simulink model "part1_2024a_Audun"  (R2024a)
settings: Solver=VariableStepAuto  StartTime=0.0  StopTime=50  RelTol=1e-3
undefined symbols (not defined in the file or in its folder): alpha, C_pitch, C_roll, C_yaw, Cx, Cy, Cz, Hoerner, magnitude, thrusters, vessel
libraries: marine_gnc x3, marine_hydro x1, simulink x1
settings Model: Creator=jonbjor  LastModifiedBy=audun
settings SolverCC: AlgebraicLoopSolver=TrustRegion
settings DataIOCC: ReturnWorkspaceOutputs=off
settings DebuggingCC: UnconnectedInputMsg=warning  UnconnectedOutputMsg=warning  UnconnectedLineMsg=warning  ArithmeticOperatorsInVariantConditions=warning
settings ModelReferenceCC: EnableRefExpFcnMdlSchedulingChecks=on
settings SFSimCC: SimUseLocalCustomCode=off  CustomCodeUndefinedFunction=UseInterfaceOnly
settings RTWCC: RTWUseLocalCustomCode=off  GPUComputeCapability=3.5  DLArmComputeVersion=19.05

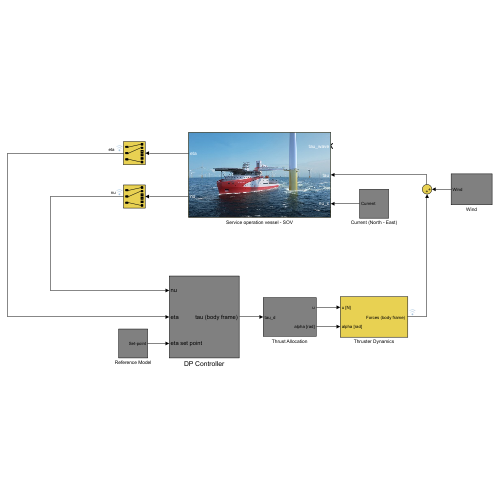
[thumbnail: Simulink's stored preview of the top-level diagram]
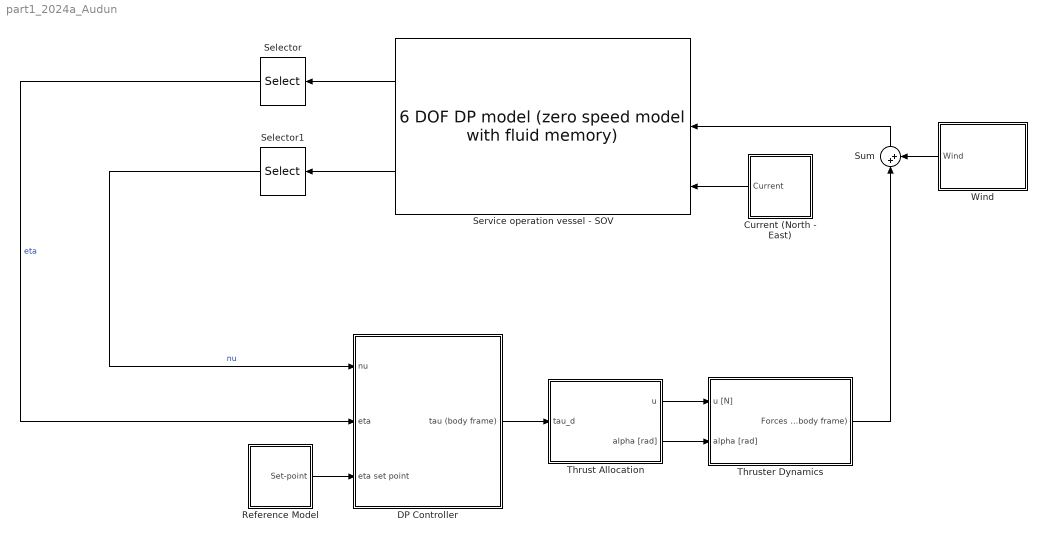
== system part1_2024a_Audun ==
  Current (North - East) : Subsystem
  DP Controller : Subsystem
  Reference Model : Subsystem
  Selector : Selector  InputPortWidth=6  IndexOptions=Index vector (dialog)  Indices=[1 2 6]  OutputSizes=1
  Selector1 : Selector  InputPortWidth=6  IndexOptions=Index vector (dialog)  Indices=[1 2 6]  OutputSizes=1
  Service operation vessel - SOV : marine_hydro/Hydro Library/6 DOF DP model  (zero speed model with fluid memory)  ABC=vesselABC  rho=1025  Axc=0.9*vessel.main.T*vessel.main.B  Ayc=0.9*vessel.main.T*vessel.main.Lpp  CX=1  CY_2D=Hoerner(vessel.main.B,vessel.main.T)  Bv=vessel.Bv  mask(6 DOF zero speed model){}
      link override "Integrator1 ": InitialCondition=nu0
      link override Integrator2: InitialCondition=eta0
      settings: SourceProductName=MSS Hydro
      mask Display:
      | image('SOV.jpg');
      | color('white'); port_label('output', 1, 'eta')
      | color('white'); port_label('output', 2, 'nu')
      | color('white'); port_label('input', 1, 'tau_wave')
      | color('white'); port_label('input', 2, 'tau')
      | color('white'); port_label('input', 3, 'nu_c')
  Sum : Sum  Inputs=|++
  Thrust Allocation : Subsystem
  Thruster Dynamics : Subsystem  mask{thrusterfault=off}
      mask prompts: thrusterfault "Fault on thruster #2 and #4?"
  Wind : Subsystem
  wires:
  Current (North - East)/1(Current) -> Service operation vessel - SOV/3
  Thruster Dynamics/1("Forces (body frame) ") -> Sum/1
  Service operation vessel - SOV/1 -> Selector/1
  Service operation vessel - SOV/2 -> Selector1/1
  Reference Model/1(Set-point) -> DP Controller/3(eta set point)
  Selector/1 -> DP Controller/2(eta)  "eta"
  Selector1/1 -> DP Controller/1(nu)  "nu"
  Thrust Allocation/1(u) -> Thruster Dynamics/1(u [N])
  Thrust Allocation/2(alpha [rad]) -> Thruster Dynamics/2(alpha [rad])
  DP Controller/1(tau (body frame)) -> Thrust Allocation/1(tau_d)
  Wind/1(Wind) -> Sum/2
  Sum/1 -> Service operation vessel - SOV/2

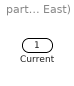
== system part1_2024a_Audun/Current (North - East) ==
  Current : Outport  VectorParamsAs1DForOutWhenUnconnected=off

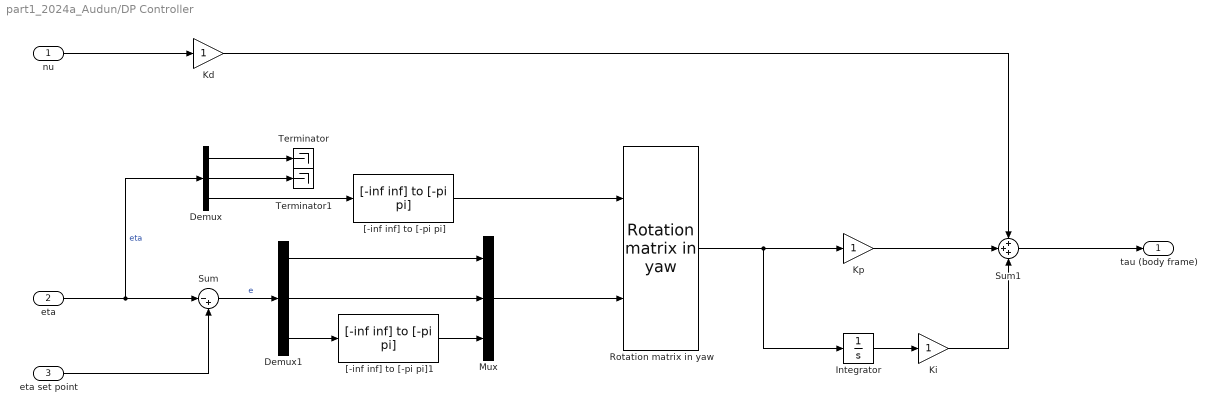
== system part1_2024a_Audun/DP Controller ==
  nu : Inport
  eta : Inport  Port=2
  eta set point : Inport  Port=3
  Demux : Demux  Outputs=3
  Demux1 : Demux  Outputs=3
  Integrator : Integrator
  Kd : Gain
  Ki : Gain
  Kp : Gain
  Mux : Mux  Inputs=3
  "Rotation matrix in yaw " : marine_gnc/Models/ Kinematics/Rotation matrix in yaw 
      settings: SourceProductName=MSS GNC
  Sum : Sum  Inputs=|-+
  Sum1 : Sum  Inputs=+++
  Terminator : Terminator
  Terminator1 : Terminator
  "[-inf inf] to [-pi pi]" : marine_gnc/Utilities/Math Operations/[-inf inf] to [-pi pi]
      settings: SourceProductName=MSS GNC
  "[-inf inf] to [-pi pi]1" : marine_gnc/Utilities/Math Operations/[-inf inf] to [-pi pi]
      settings: SourceProductName=MSS GNC
  tau (body frame) : Outport  VectorParamsAs1DForOutWhenUnconnected=off
  wires:
  eta set point/1 -> Sum/2
  eta/1 -> Demux/1, Sum/1  "eta"
  Sum/1 -> Demux1/1  "e"
  nu/1 -> Kd/1
  Demux/1 -> Terminator/1
  Demux/2 -> Terminator1/1
  Demux/3 -> "[-inf inf] to [-pi pi]"/1
  "[-inf inf] to [-pi pi]"/1 -> "Rotation matrix in yaw "/1
  Demux1/2 -> Mux/2
  Demux1/3 -> "[-inf inf] to [-pi pi]1"/1
  Demux1/1 -> Mux/1
  Mux/1 -> "Rotation matrix in yaw "/2
  "[-inf inf] to [-pi pi]1"/1 -> Mux/3
  "Rotation matrix in yaw "/1 -> Integrator/1, Kp/1
  Integrator/1 -> Ki/1
  Ki/1 -> Sum1/3
  Kp/1 -> Sum1/2
  Kd/1 -> Sum1/1
  Sum1/1 -> tau (body frame)/1

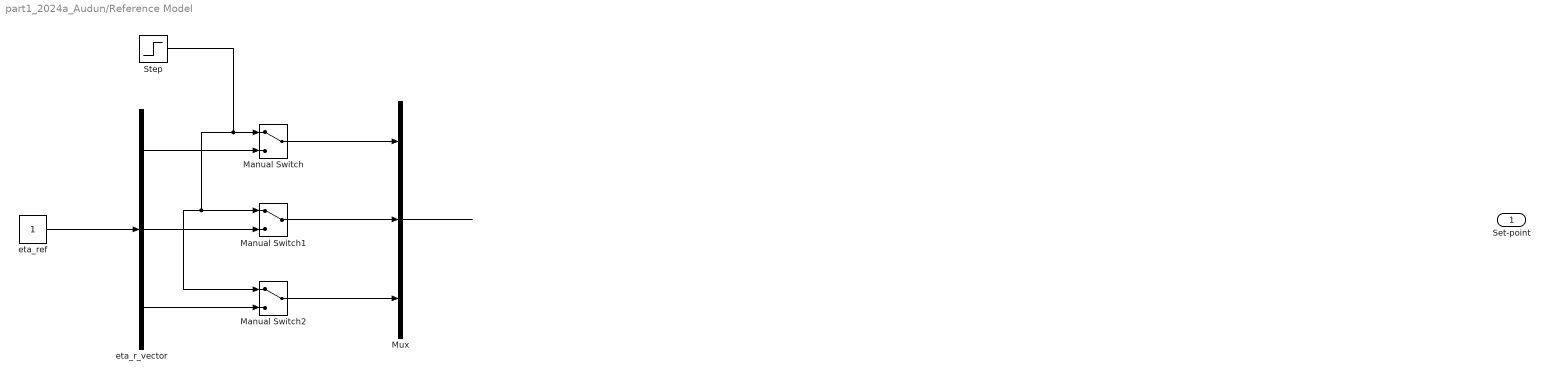
== system part1_2024a_Audun/Reference Model ==
  Manual Switch : ManualSwitch
  Manual Switch1 : ManualSwitch
  Manual Switch2 : ManualSwitch
  Mux : Mux  Inputs=3
  Step : Step  SampleTime=0
  eta_r_vector : Demux  Outputs=3
  eta_ref : Constant
  Set-point : Outport  VectorParamsAs1DForOutWhenUnconnected=off
  wires:
  ? -> Set-point/1
  eta_ref/1 -> eta_r_vector/1
  eta_r_vector/1 -> Manual Switch/2
  eta_r_vector/2 -> Manual Switch1/2
  eta_r_vector/3 -> Manual Switch2/2
  Step/1 -> Manual Switch2/1, Manual Switch1/1, Manual Switch/1
  Manual Switch/1 -> Mux/1
  Manual Switch1/1 -> Mux/2
  Manual Switch2/1 -> Mux/3
  Mux/1 -> ?

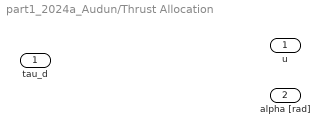
== system part1_2024a_Audun/Thrust Allocation ==
  tau_d : Inport
  u : Outport  VectorParamsAs1DForOutWhenUnconnected=off
  alpha [rad] : Outport  Port=2  VectorParamsAs1DForOutWhenUnconnected=off

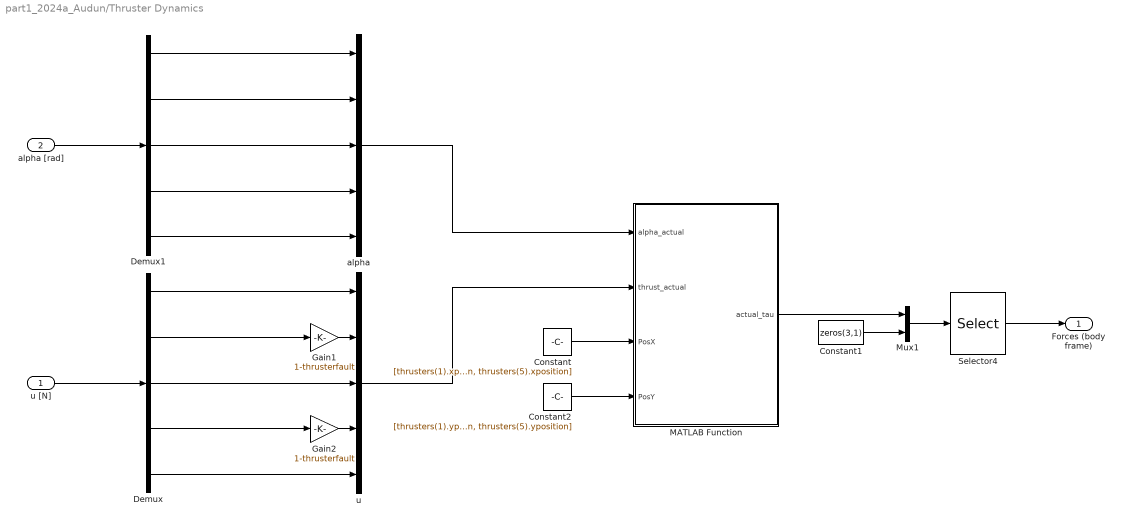
== system part1_2024a_Audun/Thruster Dynamics ==
  u [N] : Inport
  alpha [rad] : Inport  Port=2
  Constant : Constant  Value=[thrusters(1).xposition, thrusters(2).xposition, thrusters(3).xposition, thrusters(4).xposition, thrusters(5).xposition]
  Constant1 : Constant  Value=zeros(3,1)
  Constant2 : Constant  Value=[thrusters(1).yposition, thrusters(2).yposition, thrusters(3).yposition, thrusters(4).yposition, thrusters(5).yposition]
  Demux : Demux  Outputs=5
  Demux1 : Demux  Outputs=5
  Gain1 : Gain  Gain=1-thrusterfault
  Gain2 : Gain  Gain=1-thrusterfault
  MATLAB Function : MATLAB Function  TreatAsAtomicUnit=on
  Mux1 : Mux  Inputs=2
  Selector4 : Selector  InputPortWidth=6  IndexOptions=Index vector (dialog)  Indices=[1 2 4 5 6 3]  OutputSizes=1
  alpha : Mux  Inputs=5
  u : Mux  Inputs=5
  "Forces (body frame) " : Outport  VectorParamsAs1DForOutWhenUnconnected=off
  wires:
  Mux1/1 -> Selector4/1
  Constant1/1 -> Mux1/2
  Selector4/1 -> "Forces (body frame) "/1
  Gain1/1 -> u/2
  u [N]/1 -> Demux/1
  alpha [rad]/1 -> Demux1/1
  Constant/1 -> MATLAB Function/3(PosX)
  Constant2/1 -> MATLAB Function/4(PosY)
  u/1 -> MATLAB Function/2(thrust_actual)
  alpha/1 -> MATLAB Function/1(alpha_actual)
  MATLAB Function/1(actual_tau) -> Mux1/1
  Demux1/1 -> alpha/1
  Gain2/1 -> u/4
  Demux/1 -> u/1
  Demux/2 -> Gain1/1
  Demux/3 -> u/3
  Demux/4 -> Gain2/1
  Demux/5 -> u/5
  Demux1/2 -> alpha/2
  Demux1/4 -> alpha/4
  Demux1/5 -> alpha/5
  Demux1/3 -> alpha/3

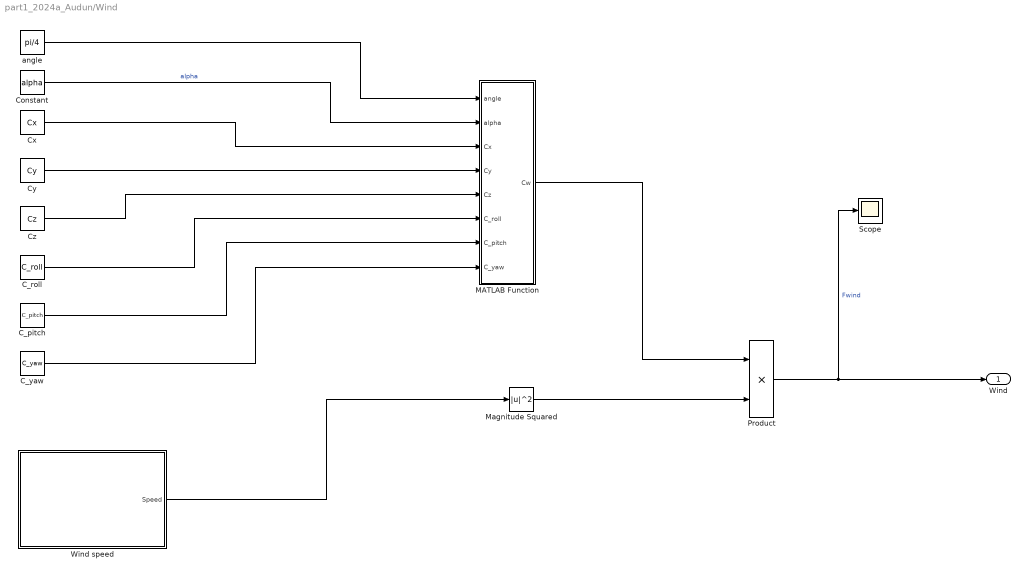
== system part1_2024a_Audun/Wind ==
  C_pitch : Constant  Value=C_pitch
  C_roll : Constant  Value=C_roll
  C_yaw : Constant  Value=C_yaw
  Constant : Constant  Value=alpha
  Cx : Constant  Value=Cx
  Cy : Constant  Value=Cy
  Cz : Constant  Value=Cz
  MATLAB Function : MATLAB Function  TreatAsAtomicUnit=on
  Magnitude Squared : Math  Operator=magnitude^2
  Product : Product
  Scope : Scope
  Wind speed : Subsystem
  angle : Constant  Value=pi/4
  Wind : Outport  VectorParamsAs1DForOutWhenUnconnected=off
  wires:
  Cz/1 -> MATLAB Function/5(Cz)
  Cy/1 -> MATLAB Function/4(Cy)
  Cx/1 -> MATLAB Function/3(Cx)
  C_yaw/1 -> MATLAB Function/8(C_yaw)
  C_roll/1 -> MATLAB Function/6(C_roll)
  C_pitch/1 -> MATLAB Function/7(C_pitch)
  Magnitude Squared/1 -> Product/2
  Product/1 -> Wind/1, Scope/1  "Fwind"
  MATLAB Function/1(Cw) -> Product/1
  Constant/1 -> MATLAB Function/2(alpha)  "alpha"
  Wind speed/1(Speed) -> Magnitude Squared/1
  angle/1 -> MATLAB Function/1(angle)

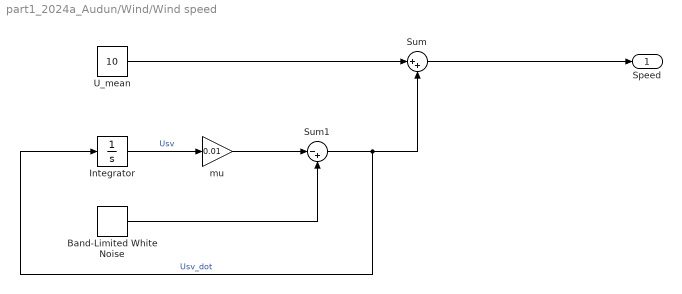
== system part1_2024a_Audun/Wind/Wind speed ==
  Band-Limited White Noise : simulink/Sources/Band-Limited White Noise  Cov=[0.1]  Ts=0.1  seed=[23341]
  Integrator : Integrator
  Sum : Sum  Inputs=|++
  Sum1 : Sum  Inputs=|-+
  U_mean : Constant  Value=10
  mu : Gain  Gain=0.01
  Speed : Outport
  wires:
  U_mean/1 -> Sum/1
  Sum/1 -> Speed/1
  mu/1 -> Sum1/1
  Integrator/1 -> mu/1  "Usv"
  Band-Limited White Noise/1 -> Sum1/2
  Sum1/1 -> Integrator/1, Sum/2  "Usv_dot"

== matlab function part1_2024a_Audun/Wind/MATLAB Function ==
  data: Cw output; angle input; alpha input; Cx input; Cy input; Cz input; C_roll input; C_pitch input; C_yaw input
function Cw = fcn(angle, alpha, Cx, Cy, Cz, C_roll, C_pitch, C_yaw)

Cw = zeros(6, 1);

index = find(abs(alpha - angle) < 1e-10);

Cw(1) = Cx(index);
Cw(2) = Cy(index);
Cw(3) = Cz(index);
Cw(4) = C_roll(index);
Cw(5) = C_pitch(index);
Cw(6) = C_yaw(index);
end

== matlab function part1_2024a_Audun/Thruster Dynamics/MATLAB Function ==
  data: alpha_actual input; thrust_actual input; actual_tau output; PosX input; PosY input
function actual_tau   = fcn(alpha_actual,thrust_actual,PosX,PosY)

    Alpha_surge =[cos(alpha_actual(1)) cos(alpha_actual(2)) cos(alpha_actual(3)) cos(alpha_actual(4)) cos(alpha_actual(5))];  
    Alpha_sway = [sin(alpha_actual(1)) sin(alpha_actual(2)) sin(alpha_actual(3)) sin(alpha_actual(4)) sin(alpha_actual(5))];
    Alpha_yaw = [sin(alpha_actual(1))*PosX(1)-cos(alpha_actual(1))*PosY(1) sin(alpha_actual(2))*PosX(2)-cos(alpha_actual(2))*PosY(2) ...
                 sin(alpha_actual(3))*PosX(3)-cos(alpha_actual(3))*PosY(3) sin(alpha_actual(4))*PosX(4)-cos(alpha_actual(4))*PosY(4) ...
                 sin(alpha_actual(5))*PosX(5)-cos(alpha_actual(5))*PosY(5)];

    actual_tau = [Alpha_surge; Alpha_sway; Alpha_yaw]*thrust_actual;
end
